simulink model "CTC2DOF_SineWave"  (R2018a)
settings: Solver=ode45  StartTime=0.0  StopTime=20  RelTol=1e-3
values from neighbouring files (symbols this model uses):
  Ki = 100    [ComputedTorqueControl_2DOF.m]
  Kp = 300    [ComputedTorqueControl_2DOF.m]
  Kv = 2*sqrt(Kp)    [ComputedTorqueControl_2DOF.m]
  omega = 0.5    [AdaptiveControl2DOF.m]    (also in ComputedTorqueControl_2DOF.m = 1)
  the1 = theta1    (= 0.959931088597)    [AdaptiveControl2DOF.m]    (also in ComputedTorqueControl_2DOF.m = 0.523598775598)
  the2 = theta2    (= -0.959931088597)    [AdaptiveControl2DOF.m]    (also in ComputedTorqueControl_2DOF.m = 0.392699081699)
  tick = 0.002    [AdaptiveControl2DOF.m]    (also in ComputedTorqueControl_2DOF.m = 0.02)
libraries: dsppolyfun x2, simulink x2
settings Model: Creator=rashe  LastModifiedBy=rashe

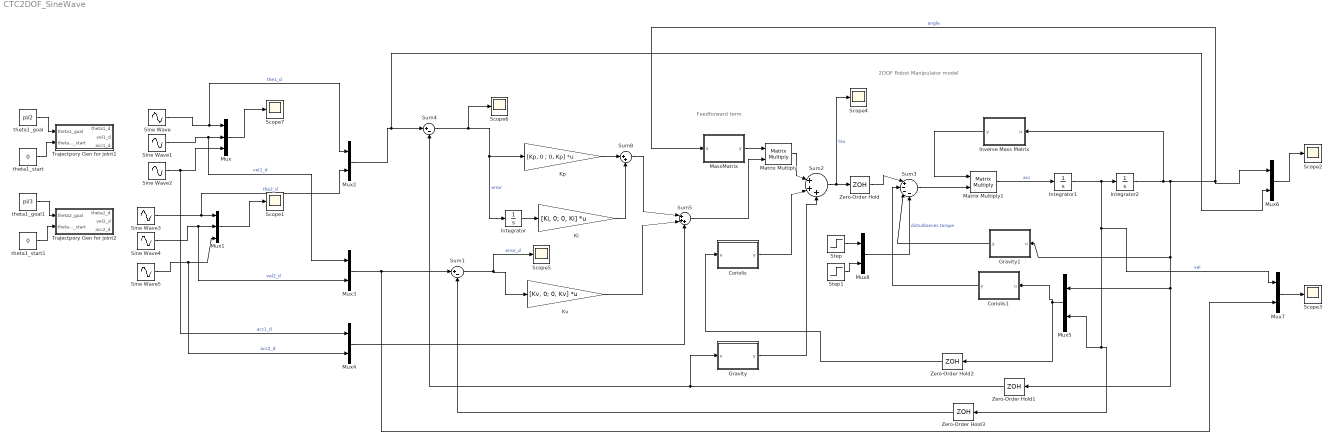
== system CTC2DOF_SineWave ==
  note: Feedforward term
  note: 2DOF Robot Manipulator model
  Coriolis : MATLAB Function  TreatAsAtomicUnit=on
  Coriolis1 : MATLAB Function  TreatAsAtomicUnit=on
  Gravity : MATLAB Function  TreatAsAtomicUnit=on
  Gravity1 : MATLAB Function  TreatAsAtomicUnit=on
  Integrator : Integrator  InitialCondition=[0; 0]
  Integrator1 : Integrator  InitialCondition=[0; 0]
  Integrator2 : Integrator  InitialCondition=[0; 0]
  Inverse Mass Matrix : MATLAB Function  TreatAsAtomicUnit=on
  Ki : Gain  Gain=[Ki, 0; 0, Ki]  Multiplication=Matrix(K*u)
  Kp : Gain  Gain=[Kp, 0 ; 0, Kp]  Multiplication=Matrix(K*u)
  Kv : Gain  Gain=[Kv, 0; 0, Kv]  Multiplication=Matrix(K*u)
  MassMatrix : MATLAB Function  TreatAsAtomicUnit=on
  Matrix Multiply : Product  Multiplication=Matrix(*)
  Matrix Multiply1 : Product  Multiplication=Matrix(*)
  Mux : Mux  Inputs=3
  Mux1 : Mux  Inputs=3
  Mux{2..8} (7 alike) : Mux  Inputs=2
  Scope{1..7} (7 alike) : Scope
  Sine Wave : Sin  Amplitude=the1  Frequency=omega  SampleTime=tick
  Sine Wave1 : Sin  Amplitude=the1*omega  Frequency=omega  Phase=pi/2  SampleTime=tick
  Sine Wave2 : Sin  Amplitude=-the1*omega  Frequency=omega  SampleTime=tick
  Sine Wave3 : Sin  Amplitude=the2  Frequency=omega  SampleTime=tick
  Sine Wave4 : Sin  Amplitude=the2*omega  Frequency=omega  Phase=pi/2  SampleTime=tick
  Sine Wave5 : Sin  Amplitude=-the2*omega  Frequency=omega  SampleTime=tick
  Step : Step  Time=10  After=0  SampleTime=0
  Step1 : Step  Time=15  After=0  SampleTime=0
  Sum1 : Sum  Inputs=|+-
  Sum2 : Sum  Inputs=|+++
  Sum3 : Sum  Inputs=|+---
  Sum4 : Sum  Inputs=|+-
  Sum5 : Sum  Inputs=|+++
  Sum8 : Sum  Inputs=|++
  Trajectpory Gen for joint1 : Subsystem
  Trajectpory Gen for joint2 : Subsystem
  Zero-Order Hold{,1..3} (4 alike) : ZeroOrderHold  SampleTime=tick
  theta1_goal : Constant  Value=pi/2  SampleTime=tick
  theta1_goal1 : Constant  Value=pi/3  SampleTime=tick
  theta1_start : Constant  Value=0  SampleTime=tick
  theta1_start1 : Constant  Value=0  SampleTime=tick
  wires:
  theta1_goal/1 -> Trajectpory Gen for joint1/1(theta1_goal)
  theta1_start/1 -> Trajectpory Gen for joint1/2(theta1_start)
  Mux/1 -> Scope7/1
  theta1_start1/1 -> Trajectpory Gen for joint2/2(theta2_start)
  theta1_goal1/1 -> Trajectpory Gen for joint2/1(theta2_goal)
  Mux1/1 -> Scope1/1
  Inverse Mass Matrix/1(y) -> Matrix Multiply1/1
  Integrator1/1 -> Mux7/1, Zero-Order Hold3/1, Mux5/2, Integrator2/1  "vel"
  Sum3/1 -> Matrix Multiply1/2
  Coriolis1/1(y) -> Sum3/2
  Coriolis/1(y) -> Sum2/2
  Gravity/1(y) -> Sum2/3
  Gravity1/1(y) -> Sum3/3
  Sum1/1 -> Scope5/1, Kv/1  "error_d"
  Sum8/1 -> Sum5/1
  Kv/1 -> Sum5/2
  Matrix Multiply/1 -> Sum2/1
  Sum2/1 -> Scope4/1, Zero-Order Hold/1  "tau"
  Mux5/1 -> Zero-Order Hold2/1, Coriolis1/1(u)
  Sum4/1 -> Scope6/1, Integrator/1, Kp/1  "error"
  Sum5/1 -> Matrix Multiply/2
  Kp/1 -> Sum8/1
  Matrix Multiply1/1 -> Integrator1/1  "acc"
  MassMatrix/1(y) -> Matrix Multiply/1
  Integrator2/1 -> MassMatrix/1(u), Mux6/1, Zero-Order Hold1/1, Mux5/1, Gravity1/1(u), Inverse Mass Matrix/1(u)  "angle"
  Ki/1 -> Sum8/2
  Integrator/1 -> Ki/1
  Mux2/1 -> Mux6/2, Sum4/1
  Mux3/1 -> Mux7/2, Sum1/1
  Mux4/1 -> Sum5/3
  Mux6/1 -> Scope2/1
  Mux7/1 -> Scope3/1
  Zero-Order Hold1/1 -> Gravity/1(u), Sum4/2
  Zero-Order Hold2/1 -> Coriolis/1(u)
  Zero-Order Hold3/1 -> Sum1/2
  Zero-Order Hold/1 -> Sum3/1
  Step/1 -> Mux8/1
  Step1/1 -> Mux8/2
  Sine Wave/1 -> Mux2/1, Mux/1  "the1_d"
  Sine Wave1/1 -> Mux3/1, Mux/2  "vel1_d"
  Sine Wave2/1 -> Mux4/1, Mux/3  "acc1_d"
  Sine Wave3/1 -> Mux2/2, Mux1/1  "the2_d"
  Sine Wave4/1 -> Mux3/2, Mux1/2  "vel2_d"
  Sine Wave5/1 -> Mux4/2, Mux1/3  "acc2_d"
  Mux8/1 -> Sum3/4  "disturbances torque"

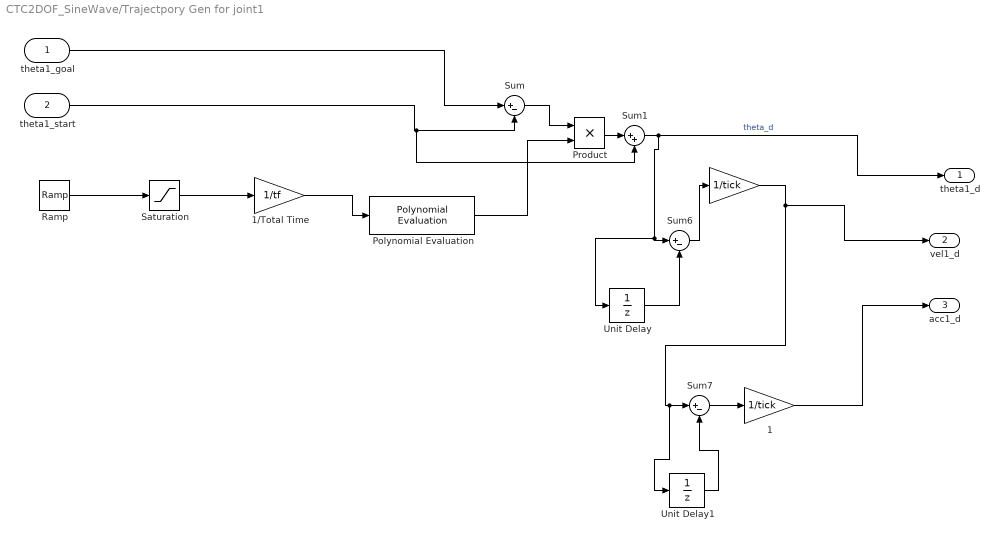
== system CTC2DOF_SineWave/Trajectpory Gen for joint1 ==
  theta1_goal : Inport
  theta1_start : Inport  Port=2
  " " : Gain  Gain=1/tick
  " 1" : Gain  Gain=1/tick
  "1/Total Time " : Gain  Gain=1/tf
  Polynomial Evaluation : dsppolyfun/Polynomial Evaluation  useConstCoeffs=on  constCoeffs=[6 -15 10 0 0 0]
      settings: SourceProductName=DSP System Toolbox  SourceProductBaseCode=DS
  Product : Product
  Ramp : simulink/Sources/Ramp  slope=1  start=0  InitialOutput=0
  Saturation : Saturate  UpperLimit=tf  LowerLimit=-tf
  Sum : Sum  Inputs=|+-
  Sum1 : Sum  Inputs=|++
  Sum6 : Sum  Inputs=|+-
  Sum7 : Sum  Inputs=|+-
  Unit Delay : UnitDelay  SampleTime=tick
  Unit Delay1 : UnitDelay  SampleTime=tick
  theta1_d : Outport
  vel1_d : Outport  Port=2
  acc1_d : Outport  Port=3
  wires:
  Sum6/1 -> " "/1
  Sum/1 -> Product/1
  Sum1/1 -> theta1_d/1, Unit Delay/1, Sum6/1  "theta_d"
  " "/1 -> vel1_d/1, Unit Delay1/1, Sum7/1
  Polynomial Evaluation/1 -> Product/2
  Sum7/1 -> " 1"/1
  Unit Delay1/1 -> Sum7/2
  Ramp/1 -> Saturation/1
  "1/Total Time "/1 -> Polynomial Evaluation/1
  Saturation/1 -> "1/Total Time "/1
  Unit Delay/1 -> Sum6/2
  Product/1 -> Sum1/1
  " 1"/1 -> acc1_d/1
  theta1_goal/1 -> Sum/1
  theta1_start/1 -> Sum1/2, Sum/2

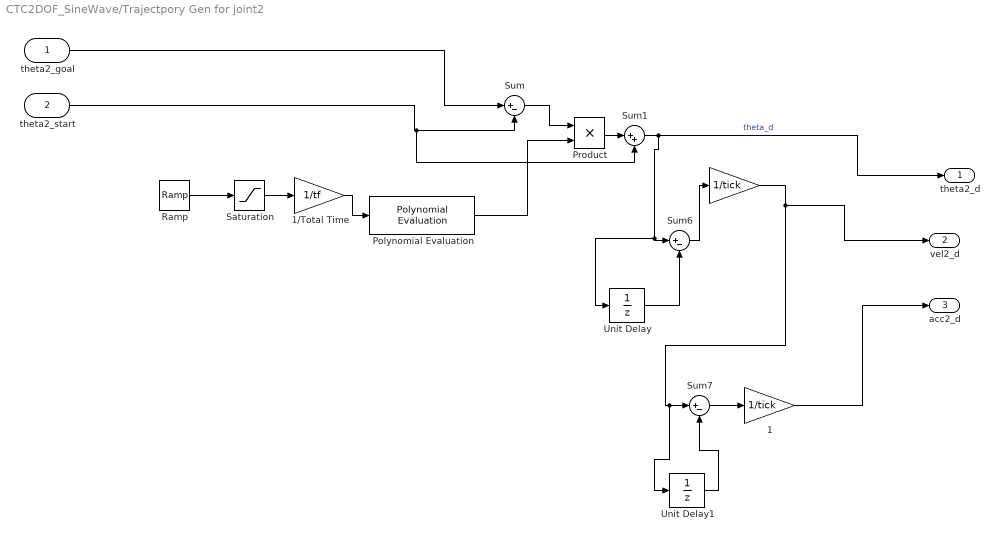
== system CTC2DOF_SineWave/Trajectpory Gen for joint2 ==
  theta2_goal : Inport
  theta2_start : Inport  Port=2
  " " : Gain  Gain=1/tick
  " 1" : Gain  Gain=1/tick
  "1/Total Time " : Gain  Gain=1/tf
  Polynomial Evaluation : dsppolyfun/Polynomial Evaluation  useConstCoeffs=on  constCoeffs=[6 -15 10 0 0 0]
      settings: SourceProductName=DSP System Toolbox  SourceProductBaseCode=DS
  Product : Product
  Ramp : simulink/Sources/Ramp  slope=1  start=0  InitialOutput=0
  Saturation : Saturate  UpperLimit=tf  LowerLimit=-tf
  Sum : Sum  Inputs=|+-
  Sum1 : Sum  Inputs=|++
  Sum6 : Sum  Inputs=|+-
  Sum7 : Sum  Inputs=|+-
  Unit Delay : UnitDelay  SampleTime=tick
  Unit Delay1 : UnitDelay  SampleTime=tick
  theta2_d : Outport
  vel2_d : Outport  Port=2
  acc2_d : Outport  Port=3
  wires:
  Sum6/1 -> " "/1
  Sum/1 -> Product/1
  Sum1/1 -> theta2_d/1, Unit Delay/1, Sum6/1  "theta_d"
  " "/1 -> vel2_d/1, Unit Delay1/1, Sum7/1
  Polynomial Evaluation/1 -> Product/2
  Sum7/1 -> " 1"/1
  Unit Delay1/1 -> Sum7/2
  Ramp/1 -> Saturation/1
  "1/Total Time "/1 -> Polynomial Evaluation/1
  Saturation/1 -> "1/Total Time "/1
  Unit Delay/1 -> Sum6/2
  Product/1 -> Sum1/1
  " 1"/1 -> acc2_d/1
  theta2_goal/1 -> Sum/1
  theta2_start/1 -> Sum1/2, Sum/2

== matlab function CTC2DOF_SineWave/Coriolis ==
  data: u input; y output
function y = V(u)

the1 = u(1);
the2 = u(2);

vel1 = u(3);
vel2 = u(4);

m1 = 0.233;   %kg
m2 = 0.2;
l1 = 0.192;
l2 = 0.185;
L1 = 0.27;
L2 = 0.23;
g = 9.81;

I1 = (1/3)*m1*l1^2;
I2 = (1/3)*m2*l2^2;


V11 = -m2*L1*l2*sin(the2)*(vel1*vel2 + 0.5*vel2^2);
V21 = 0.5*m2*L1*l2*sin(the2)*vel1^2;


y = [V11;V21];

== matlab function CTC2DOF_SineWave/MassMatrix ==
  data: u input; y output
function y = MassMatrix(u)
the1 = u(1);
the2 = u(2);

m1 = 0.233;   %kg
m2 = 0.2;
l1 = 0.192;
l2 = 0.185;
L1 = 0.27;
L2 = 0.23;
g = 9.81;

I1 = (1/3)*m1*l1^2;
I2 = (1/3)*m2*l2^2;

M11 = m1*l1^2 + m2*(L1^2 + l2^2 + L1*l2*cos(the2)) + I1 + I2;
M12 = m2*(l2^2 + L1*l2*cos(the2)) + I2;
M21 = m2*(l2^2 + L1*l2*cos(the2)) + I2;
M22 = m2*l2^2 + I2;



y = [M11, M12; M21, M22];

== matlab function CTC2DOF_SineWave/Inverse Mass Matrix ==
  data: u input; y output
function y = INVMass(u)

the1 = u(1);
the2 = u(2);

m1 = 0.233;   %kg
m2 = 0.2;
l1 = 0.23;    % chagne the parameter value for make an imperfect model
l2 = 0.17;    % chagne the parameter value for make an imperfect model
L1 = 0.3;     % chagne the parameter value for make an imperfect model
%l1 = 0.192;  % This is perferct parameter for perfect model
%l2 = 0.185; % This is perferct parameter for perfect model
%L1 = 0.27;   % This is perferct parameter for perfect model
L2 = 0.23;
g = 9.81;

I1 = (1/3)*m1*l1^2;
I2 = (1/3)*m2*l2^2;

M11 = m1*l1^2 + m2*(L1^2 + l2^2 + L1*l2*cos(the2)) + I1 + I2;
M12 = m2*(l2^2 + L1*l2*cos(the2)) + I2;
M21 = m2*(l2^2 + L1*l2*cos(the2)) + I2;
M22 = m2*l2^2 + I2;

coef = 1/(M11*M22 - M12*M21);
invM = coef*[M22, -M12; -M21, M11];

y = invM;

== matlab function CTC2DOF_SineWave/Gravity ==
  data: u input; y output
function y = G(u)

the1 = u(1);
the2 = u(2);

m1 = 0.233;   %kg
m2 = 0.2;
l1 = 0.192;
l2 = 0.185;
L1 = 0.27;
L2 = 0.23;
g = 9.81;

I1 = (1/3)*m1*l1^2;
I2 = (1/3)*m2*l2^2;

G11 = m1*g*l1*cos(the1) + m2*g*L1*cos(the1) + m2*g*l2*cos(the1+the2);
G21 = m2*g*l2*cos(the1+the2);

y = [G11;G21];

== matlab function CTC2DOF_SineWave/Coriolis1 ==
  data: u input; y output
function y = V(u)

the1 = u(1);
the2 = u(2);

vel1 = u(3);
vel2 = u(4);

m1 = 0.233;   %kg
m2 = 0.2;
l1 = 0.23;    % chagne the parameter value for make an imperfect model
l2 = 0.17;    % chagne the parameter value for make an imperfect model
L1 = 0.3;     % chagne the parameter value for make an imperfect model
%l1 = 0.192;  % This is perferct parameter for perfect model
%l2 = 0.185; % This is perferct parameter for perfect model
%L1 = 0.27;   % This is perferct parameter for perfect model
L2 = 0.23;
g = 9.81;

I1 = (1/3)*m1*l1^2;
I2 = (1/3)*m2*l2^2;



V11 = -m2*L1*l2*sin(the2)*(vel1*vel2 + 0.5*vel2^2);
V21 = 0.5*m2*L1*l2*sin(the2)*vel1^2;


y = [V11;V21];

== matlab function CTC2DOF_SineWave/Gravity1 ==
  data: u input; y output
function y = G(u)

the1 = u(1);
the2 = u(2);

m1 = 0.233;   %kg
m2 = 0.2;
l1 = 0.23;    % chagne the parameter value for make an imperfect model
l2 = 0.17;    % chagne the parameter value for make an imperfect model
%l1 = 0.192;  % This is perferct parameter for perfect model
%l2 = 0.185; % This is perferct parameter for perfect model
L1 = 0.27;
L2 = 0.23;
g = 9.81;

I1 = (1/3)*m1*l1^2;
I2 = (1/3)*m2*l2^2;

G11 = m1*g*l1*cos(the1) + m2*g*L1*cos(the1) + m2*g*l2*cos(the1+the2);
G21 = m2*g*l2*cos(the1+the2);

y = [G11;G21];
